simulink model "fivestatespace"  (R2020b)
settings: Solver=VariableStepAuto  StartTime=0.0  StopTime=10.00  RelTol=1e-3
values from neighbouring files (symbols this model uses):
  Beq = 0.2963    [milestone1constants.m]
  Jeq = 0.01802    [milestone1constants.m]
  Kb = 2.2179e-3    (= 0.0022179)    [milestone1constants.m]
  Keq = 0.74    [milestone1constants.m]
  Nmotor = 333.6375    [milestone1constants.m]
  p = 0.037    [milestone1constants.m]
  ra = 7.4    [milestone1constants.m]
  step_time = 5    [milestone1constants.m]
  theta_i = 0    [milestone1constants.m]
  u_l_f = 3    [milestone1constants.m]
  u_l_i = 5    [milestone1constants.m]
  u_r_f = 9    [milestone1constants.m]
  u_r_i = 10    [milestone1constants.m]
  wl_i = 0    [milestone1constants.m]
  Wr = 0.18    [milestone1constants.m]
  wr_i = 0    [milestone1constants.m]
  x_i = 0    [milestone1constants.m]
  y_i = 0    [milestone1constants.m]
settings Model: Creator=oliviaball  LastModifiedBy=oliviaball
settings DataIOCC: ReturnWorkspaceOutputs=off
settings DebuggingCC: ArithmeticOperatorsInVariantConditions=warning
settings SFSimCC: CustomCodeUndefinedFunction=UseInterfaceOnly

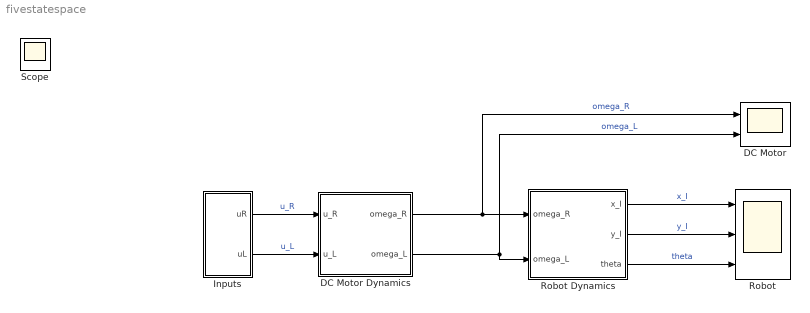
== system fivestatespace ==
  DC Motor : Scope  NumInputPorts=2
  DC Motor Dynamics : Subsystem
  Inputs : Subsystem
  Robot : Scope  NumInputPorts=3
  Robot Dynamics : Subsystem
  Scope : Scope
  wires:
  Inputs/1(uR) -> DC Motor Dynamics/1(u_R)  "u_R"
  Inputs/2(uL) -> DC Motor Dynamics/2(u_L)  "u_L"
  DC Motor Dynamics/1(omega_R) -> DC Motor/1, Robot Dynamics/1(omega_R)  "omega_R"
  DC Motor Dynamics/2(omega_L) -> DC Motor/2, Robot Dynamics/2(omega_L)  "omega_L"
  Robot Dynamics/1(x_I) -> Robot/1  "x_I"
  Robot Dynamics/2("y_I ") -> Robot/2  "y_I"
  Robot Dynamics/3(theta) -> Robot/3  "theta"

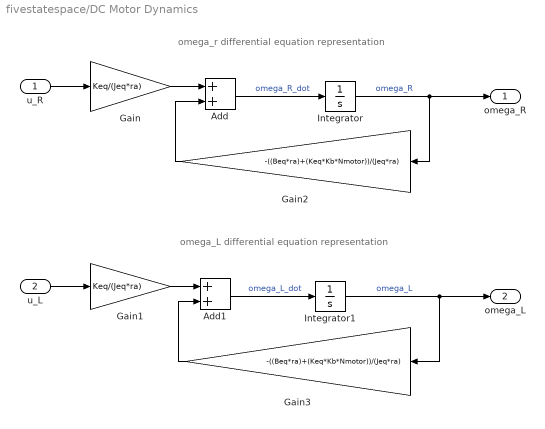
== system fivestatespace/DC Motor Dynamics ==
  note: omega_L differential equation representation
  note: omega_r differential equation representation
  u_R : Inport
  u_L : Inport  Port=2
  Add : Sum
  Add1 : Sum
  Gain : Gain  Gain=Keq/(Jeq*ra)
  Gain1 : Gain  Gain=Keq/(Jeq*ra)
  Gain2 : Gain  Gain=-((Beq*ra)+(Keq*Kb*Nmotor))/(Jeq*ra)
  Gain3 : Gain  Gain=-((Beq*ra)+(Keq*Kb*Nmotor))/(Jeq*ra)
  Integrator : Integrator  InitialCondition=wr_i
  Integrator1 : Integrator  InitialCondition=wl_i
  omega_R : Outport  VectorParamsAs1DForOutWhenUnconnected=off
  omega_L : Outport  Port=2  VectorParamsAs1DForOutWhenUnconnected=off
  wires:
  u_R/1 -> Gain/1
  Gain/1 -> Add/1
  Add/1 -> Integrator/1  "omega_R_dot"
  Integrator/1 -> omega_R/1, Gain2/1  "omega_R"
  Gain2/1 -> Add/2
  Gain3/1 -> Add1/2
  Add1/1 -> Integrator1/1  "omega_L_dot"
  Gain1/1 -> Add1/1
  Integrator1/1 -> omega_L/1, Gain3/1  "omega_L"
  u_L/1 -> Gain1/1

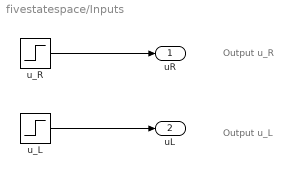
== system fivestatespace/Inputs ==
  note: Output u_R
  note: Output u_L
  u_L : Step  Time=step_time  Before=u_l_i  After=u_l_f  SampleTime=0
  u_R : Step  Time=step_time  Before=u_r_i  After=u_r_f  SampleTime=0
  uR : Outport  VectorParamsAs1DForOutWhenUnconnected=off
  uL : Outport  Port=2  VectorParamsAs1DForOutWhenUnconnected=off
  wires:
  u_L/1 -> uL/1
  u_R/1 -> uR/1

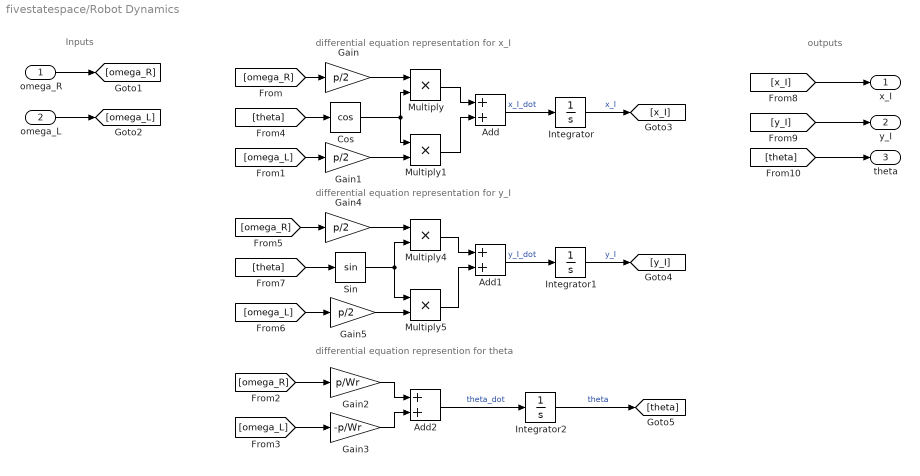
== system fivestatespace/Robot Dynamics ==
  note: Inputs
  note: outputs
  note: differential equation representation for y_I
  note: differential equation represention for theta
  note: differential equation representation for x_I
  omega_R : Inport
  omega_L : Inport  Port=2
  Add : Sum
  Add1 : Sum
  Add2 : Sum
  Cos : Trigonometry  Operator=cos
  Gain{,1,4..5} (4 alike) : Gain  Gain=p/2
  Gain2 : Gain  Gain=p/Wr
  Gain3 : Gain  Gain=-p/Wr
  Integrator : Integrator  InitialCondition=x_i
  Integrator1 : Integrator  InitialCondition=y_i
  Integrator2 : Integrator  InitialCondition=theta_i
  Multiply{,1,4..5} (4 alike) : Product
  Sin : Trigonometry
  x_I : Outport  VectorParamsAs1DForOutWhenUnconnected=off
  "y_I " : Outport  Port=2  VectorParamsAs1DForOutWhenUnconnected=off
  theta : Outport  Port=3  VectorParamsAs1DForOutWhenUnconnected=off
  wires:
  omega_R/1 -> [omega_R]
  omega_L/1 -> [omega_L]
  [omega_L] -> Gain5/1
  Multiply5/1 -> Add1/2
  [omega_R] -> Gain4/1
  Integrator/1 -> [x_I]  "x_I"
  [theta] -> theta/1
  Gain/1 -> Multiply/1
  Integrator1/1 -> [y_I]  "y_I"
  Multiply4/1 -> Add1/1
  Add2/1 -> Integrator2/1  "theta_dot"
  Add1/1 -> Integrator1/1  "y_I_dot"
  Multiply1/1 -> Add/2
  Gain4/1 -> Multiply4/1
  Multiply/1 -> Add/1
  Gain2/1 -> Add2/1
  [y_I] -> "y_I "/1
  [x_I] -> x_I/1
  Gain5/1 -> Multiply5/2
  [omega_L] -> Gain1/1
  [theta] -> Cos/1
  Gain1/1 -> Multiply1/2
  [theta] -> Sin/1
  [omega_L] -> Gain3/1
  Add/1 -> Integrator/1  "x_I_dot"
  Sin/1 -> Multiply5/1, Multiply4/2
  Integrator2/1 -> [theta]  "theta"
  [omega_R] -> Gain/1
  Cos/1 -> Multiply1/1, Multiply/2
  [omega_R] -> Gain2/1
  Gain3/1 -> Add2/2
